simulink model "projekt_n"  (R2023b)
settings: Solver=ode3  StartTime=0.0  StopTime=4  FixedStep=1e-4  RelTol=1e-3
values from neighbouring files (symbols this model uses):
  B = J*Rt/psi_en^2    (= 0.516019950154)    [dane.m]    (also in kod.m = 0.258009975077; naped.m = 0.0938218091189)
  I_N = 85    [kod.m]
  J = 11*Js    (= 8.25)    [dane.m]    (also in kod.m; naped.m = 3)
  K_P = (1.5*U_N)/10    (= 34.5)    [kod.m]
  K_T = (10)/(1.2*w_N)    (= 0.113682102208)    [kod.m]
  K_w = J/(2*beta*psi_e*K_T*K_z)    [kod.m]
  lambda_N = 1.8    [kod.m]
  m = T1    [kod.m]    (also in naped.m)
  P_N = 17000    [kod.m]
  psi_e = (U_N-R_t*I_N)/w_N    (= 2.844257988)    [kod.m]
  R_t = 0.253    [kod.m]
  T = Lt/Rt    (= 0.00750988142292)    [dane.m]    (also in kod.m; naped.m)
  Tr = 4*beta    (= 0.144)    [kod.m]
  U_N = 230    [kod.m]
  u_z0 = lambda_N*I_N*Y*B1/(B1-beta)    [kod.m]
  V = K_P*Y*B*beta/(R_t*(B1-beta))    [kod.m]    (also in naped.m = ((Kp*Y)/R1)*((B*beta)/(B1-beta)))
  w_N = (2*pi*n_N)/60    (= 73.3038285838)    [kod.m]
  Y = 10/(2.5*In)    (= 0.0470588235294)    [dane.m]    (also in kod.m; naped.m)
settings Model: Creator=womru  LastModifiedBy=rolni
settings DataIOCC: SaveFormat=StructureWithTime  ReturnWorkspaceOutputs=off

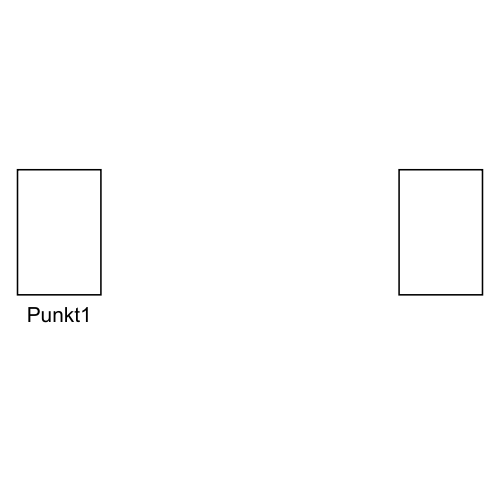
[thumbnail: Simulink's stored preview of the top-level diagram]
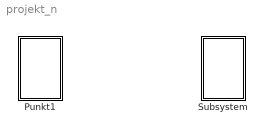
== system projekt_n ==
  Punkt1 : Subsystem
  Subsystem : Subsystem

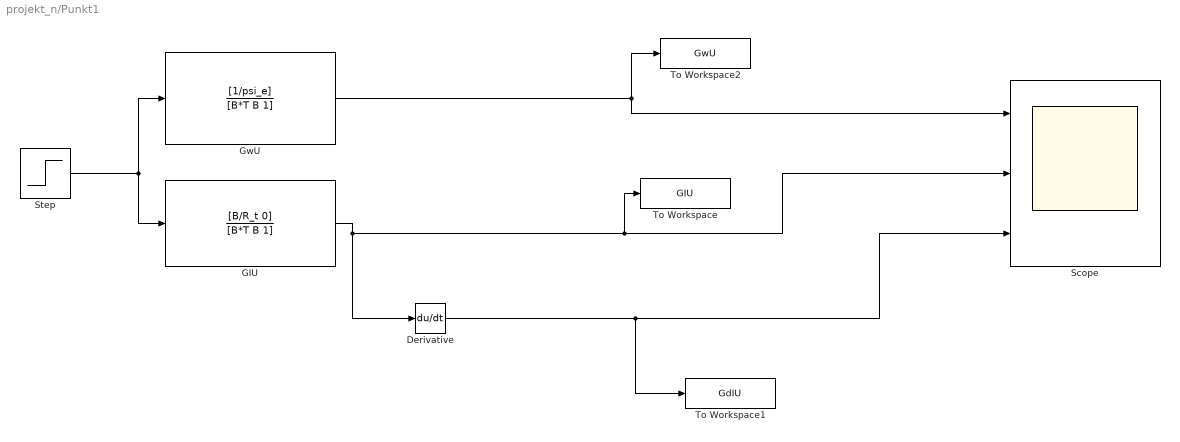
== system projekt_n/Punkt1 ==
  Derivative : Derivative
  GIU : TransferFcn  Numerator=[B/R_t 0]  Denominator=[B*T B 1]
  GwU : TransferFcn  Numerator=[1/psi_e]  Denominator=[B*T B 1]
  Scope : Scope  NumInputPorts=3
  Step : Step  Time=0  After=U_N  SampleTime=0
  To Workspace : ToWorkspace  VariableName=GIU  SaveFormat=Structure With Time  SampleTime=-1
  To Workspace1 : ToWorkspace  VariableName=GdIU  SaveFormat=Structure With Time  SampleTime=-1
  To Workspace2 : ToWorkspace  VariableName=GwU  SaveFormat=Structure With Time  SampleTime=-1
  wires:
  GIU/1 -> To Workspace/1, Scope/2, Derivative/1
  Step/1 -> GIU/1, GwU/1
  GwU/1 -> To Workspace2/1, Scope/1
  Derivative/1 -> To Workspace1/1, Scope/3

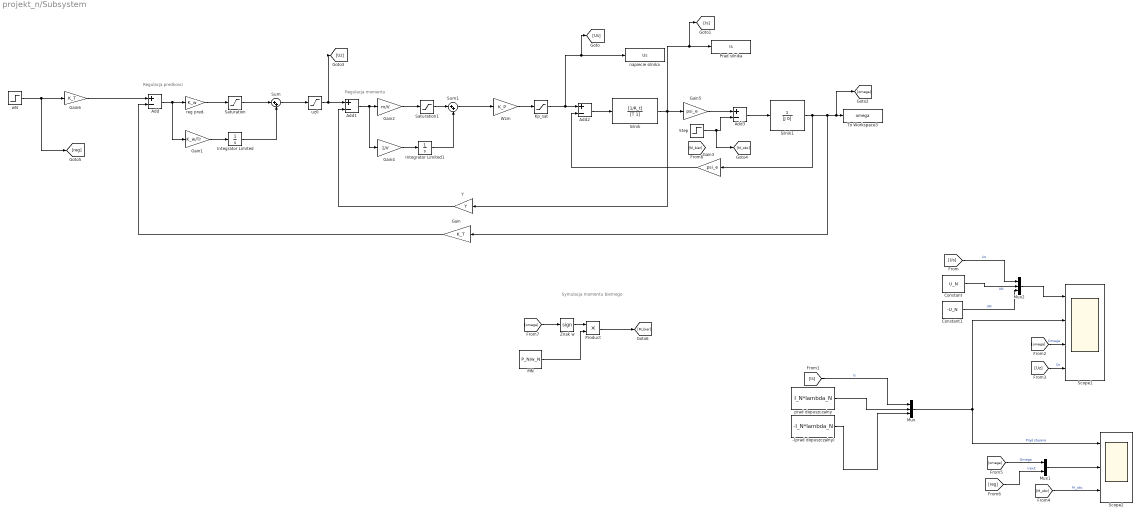
== system projekt_n/Subsystem ==
  note: Regulacja momentu
  note: Regulacja predkosci
  note: Symulacja momentu biernego
  -(prad dopuszczalny) : Constant  Value=-I_N*lambda_N
  Add{,1..3} (4 alike) : Sum  Inputs=+-
  Constant : Constant  Value=U_N
  Constant1 : Constant  Value=-U_N
  Gain : Gain  Gain=K_T
  Gain1 : Gain  Gain=K_w/Tr
  Gain2 : Gain  Gain=m/V
  Gain3 : Gain  Gain=psi_e
  Gain4 : Gain  Gain=1/V
  Gain5 : Gain  Gain=psi_e
  Gain6 : Gain  Gain=K_T
  Integrator Limited : Integrator  LimitOutput=on  UpperSaturationLimit=10  LowerSaturationLimit=-10
  Integrator Limited1 : Integrator  LimitOutput=on  UpperSaturationLimit=10  LowerSaturationLimit=-10
  Kp_sat : Saturate  UpperLimit=1.5*U_N  LowerLimit=-1.5*U_N
  MN : Constant  Value=P_N/w_N
  Mux : Mux  Inputs=3
  Mux1 : Mux  Inputs=2
  Mux2 : Mux  Inputs=3
  Prad silnika : ToWorkspace  VariableName=Is  SaveFormat=Structure With Time  SampleTime=-1
  Product : Product
  Saturation : Saturate  UpperLimit=10  LowerLimit=-10
  Saturation1 : Saturate  UpperLimit=10  LowerLimit=-10
  Scope1 : Scope  NumInputPorts=4
  Scope2 : Scope  NumInputPorts=3
  Silnik : TransferFcn  Numerator=[1/R_t]  Denominator=[T 1]
  Silnik1 : TransferFcn  Denominator=[J 0]
  Step : Step  Time=3  After=P_N/w_N  SampleTime=0
  Sum : Sum  Inputs=|++
  Sum1 : Sum  Inputs=|++
  To Workspace3 : ToWorkspace  VariableName=omega  SaveFormat=Structure With Time  SampleTime=-1
  Wzm : Gain  Gain=K_P
  Y : Gain  Gain=Y
  Znak w : Signum
  napiecie silnika : ToWorkspace  VariableName=Us  SaveFormat=Structure With Time  SampleTime=-1
  prad dopuszczalny : Constant  Value=I_N*lambda_N
  reg pred. : Gain  Gain=K_w
  uz0 : Saturate  UpperLimit=abs(u_z0)  LowerLimit=-1*abs(u_z0)
  wN : Step  Time=0  After=w_N  SampleTime=0
  wires:
  Silnik1/1 -> Gain3/1, Gain/1, [omega], To Workspace3/1
  Mux1/1 -> Scope2/2
  reg pred./1 -> Saturation/1
  Znak w/1 -> Product/1
  Gain1/1 -> Integrator Limited/1
  Gain/1 -> Add/2
  Integrator Limited1/1 -> Sum1/2
  [Is] -> Mux/1  "Is"
  Mux2/1 -> Scope1/1
  Saturation1/1 -> Sum1/1
  Kp_sat/1 -> [Us], napiecie silnika/1, Add2/1
  Gain2/1 -> Saturation1/1
  wN/1 -> [reg], Gain6/1
  Silnik/1 -> [Is], Prad silnika/1, Y/1, Gain5/1
  Constant/1 -> Mux2/2  "UN"
  prad dopuszczalny/1 -> Mux/2
  [omega] -> Scope1/3  "Omega"
  Constant1/1 -> Mux2/3  "UN"
  Sum1/1 -> Wzm/1
  Add1/1 -> Gain4/1, Gain2/1
  Gain3/1 -> Add2/2
  Mux/1 -> Scope2/1, Scope1/2  "Prąd stojana"
  -(prad dopuszczalny)/1 -> Mux/3
  Add3/1 -> Silnik1/1
  [Uz] -> Scope1/4  "Uz"
  [omega] -> Mux1/1  "Omega"
  Product/1 -> [M_bier]
  [omega] -> Znak w/1
  Sum/1 -> uz0/1
  MN/1 -> Product/2
  Saturation/1 -> Sum/1
  uz0/1 -> [Uz], Add1/1
  Gain6/1 -> Add/1
  [reg] -> Mux1/2  "input"
  [Us] -> Mux2/1  "Us"
  [M_obc] -> Scope2/3  "M_obc"
  Y/1 -> Add1/2
  Add2/1 -> Silnik/1
  Wzm/1 -> Kp_sat/1
  Add/1 -> Gain1/1, reg pred./1
  Gain5/1 -> Add3/1
  Gain4/1 -> Integrator Limited1/1
  Integrator Limited/1 -> Sum/2
  Step/1 -> [M_obc], Add3/2
